simulink model "gm_mandelbrot_fpga"  (R2019b)
settings: Solver=FixedStepDiscrete  StartTime=0.0  StopTime=33.5e-3  FixedStep=0.5*Ts  RelTol=1e-3  EnableMultiTasking=on
undefined symbols (not defined in the file or in its folder): BUTTON_CLOCK_DIV, BUTTON_DEBOUNCE, BUTTON_POLLING, LUT_BLUE, LUT_GREEN, LUT_RED, MAX_ITERATIONS, PIXEL_TIME, TRASLATION_FACTOR, Ts, VGA_HORIZONTAL_BACK_PORCH, VGA_HORIZONTAL_FRONT_PORCH, VGA_HORIZONTAL_RESOLUTION, VGA_HORIZONTAL_SYNC, VGA_VERTICAL_BACK_PORCH, VGA_VERTICAL_FRONT_PORCH, VGA_VERTICAL_RESOLUTION, VGA_VERTICAL_SYNC, ZOOM_FACTOR
libraries: simulink x132, hdlsllib x20, visionsinks x1
(part 7 of 9)

== system gm_mandelbrot_fpga/mandelbrot_top/mandelbrot_core/mandelbroot_pipeline/mandelbroot_array_instance57 ==
  stop_in : Inport  OutDataTypeStr=boolean  PortDimensions=1  SampleTime=1.35e-08
  z_in : Inport  Port=2  OutDataTypeStr=fixdt(1, 18, 15)  PortDimensions=1  SampleTime=1.35e-08
      settings: SignalType=complex
  c_in : Inport  Port=3  OutDataTypeStr=fixdt(1, 18, 15)  PortDimensions=1  SampleTime=1.35e-08
      settings: SignalType=complex
  i_in : Inport  Port=4  OutDataTypeStr=fixdt(0, 7, 0)  PortDimensions=1  SampleTime=1.35e-08
  Add : Sum
  Add1 : Sum  Inputs=+-  OutDataTypeStr=Inherit: Same as first input
  Compare To Constant : simulink/Logic and Bit Operations/Compare To Constant  relop=>=  const=4  OutDataTypeStr=boolean
  Complex to Real-Imag : ComplexToRealImag
  Constant : Constant  OutDataTypeStr=uint8  SampleTime=-1
  Data Type Conversion2 : DataTypeConversion
  Gain : Gain  Gain=2  OutDataTypeStr=Inherit: Same as input  ParamDataTypeStr=Inherit: Same as input
  Logical Operator : Logic  Operator=OR  IconShape=distinctive  AllPortsSameDT=off  OutDataTypeStr=boolean
  Product1 : Product
  Product2 : Product
  Product3 : Product
  Real-Imag to Complex : RealImagToComplex
  Sum : Sum  Inputs=|++  OutDataTypeStr=Inherit: Same as first input
  Sum1 : Sum  Inputs=|++
  Switch : Switch  Criteria=u2 ~= 0
  stop_out : Outport  VectorParamsAs1DForOutWhenUnconnected=off
  z_out : Outport  Port=2  VectorParamsAs1DForOutWhenUnconnected=off
  c_out : Outport  Port=3  VectorParamsAs1DForOutWhenUnconnected=off
  i_out : Outport  Port=4  VectorParamsAs1DForOutWhenUnconnected=off
  wires:
  i_in/1 -> Switch/1, Sum1/1
  c_in/1 -> c_out/1, Sum/2
  z_in/1 -> Complex to Real-Imag/1
  stop_in/1 -> Logical Operator/1
  Add/1 -> Compare To Constant/1
  Add1/1 -> Real-Imag to Complex/1
  Compare To Constant/1 -> Logical Operator/2
  Complex to Real-Imag/2 -> Product3/2, Product2/1, Product2/2
  Complex to Real-Imag/1 -> Product3/1, Product1/1, Product1/2
  Constant/1 -> Sum1/2
  Data Type Conversion2/1 -> z_out/1
  Gain/1 -> Real-Imag to Complex/2
  Logical Operator/1 -> stop_out/1, Switch/2
  Product1/1 -> Add1/1, Add/1
  Product2/1 -> Add1/2, Add/2
  Product3/1 -> Gain/1
  Real-Imag to Complex/1 -> Sum/1
  Sum/1 -> Data Type Conversion2/1
  Sum1/1 -> Switch/3
  Switch/1 -> i_out/1

== system gm_mandelbrot_fpga/mandelbrot_top/mandelbrot_core/mandelbroot_pipeline/mandelbroot_array_instance58 ==
  stop_in : Inport  OutDataTypeStr=boolean  PortDimensions=1  SampleTime=1.35e-08
  z_in : Inport  Port=2  OutDataTypeStr=fixdt(1, 18, 15)  PortDimensions=1  SampleTime=1.35e-08
      settings: SignalType=complex
  c_in : Inport  Port=3  OutDataTypeStr=fixdt(1, 18, 15)  PortDimensions=1  SampleTime=1.35e-08
      settings: SignalType=complex
  i_in : Inport  Port=4  OutDataTypeStr=fixdt(0, 7, 0)  PortDimensions=1  SampleTime=1.35e-08
  Add : Sum
  Add1 : Sum  Inputs=+-  OutDataTypeStr=Inherit: Same as first input
  Compare To Constant : simulink/Logic and Bit Operations/Compare To Constant  relop=>=  const=4  OutDataTypeStr=boolean
  Complex to Real-Imag : ComplexToRealImag
  Constant : Constant  OutDataTypeStr=uint8  SampleTime=-1
  Data Type Conversion2 : DataTypeConversion
  Gain : Gain  Gain=2  OutDataTypeStr=Inherit: Same as input  ParamDataTypeStr=Inherit: Same as input
  Logical Operator : Logic  Operator=OR  IconShape=distinctive  AllPortsSameDT=off  OutDataTypeStr=boolean
  Product1 : Product
  Product2 : Product
  Product3 : Product
  Real-Imag to Complex : RealImagToComplex
  Sum : Sum  Inputs=|++  OutDataTypeStr=Inherit: Same as first input
  Sum1 : Sum  Inputs=|++
  Switch : Switch  Criteria=u2 ~= 0
  stop_out : Outport  VectorParamsAs1DForOutWhenUnconnected=off
  z_out : Outport  Port=2  VectorParamsAs1DForOutWhenUnconnected=off
  c_out : Outport  Port=3  VectorParamsAs1DForOutWhenUnconnected=off
  i_out : Outport  Port=4  VectorParamsAs1DForOutWhenUnconnected=off
  wires:
  i_in/1 -> Switch/1, Sum1/1
  c_in/1 -> c_out/1, Sum/2
  z_in/1 -> Complex to Real-Imag/1
  stop_in/1 -> Logical Operator/1
  Add/1 -> Compare To Constant/1
  Add1/1 -> Real-Imag to Complex/1
  Compare To Constant/1 -> Logical Operator/2
  Complex to Real-Imag/2 -> Product3/2, Product2/1, Product2/2
  Complex to Real-Imag/1 -> Product3/1, Product1/1, Product1/2
  Constant/1 -> Sum1/2
  Data Type Conversion2/1 -> z_out/1
  Gain/1 -> Real-Imag to Complex/2
  Logical Operator/1 -> stop_out/1, Switch/2
  Product1/1 -> Add1/1, Add/1
  Product2/1 -> Add1/2, Add/2
  Product3/1 -> Gain/1
  Real-Imag to Complex/1 -> Sum/1
  Sum/1 -> Data Type Conversion2/1
  Sum1/1 -> Switch/3
  Switch/1 -> i_out/1

== system gm_mandelbrot_fpga/mandelbrot_top/mandelbrot_core/mandelbroot_pipeline/mandelbroot_array_instance59 ==
  stop_in : Inport  OutDataTypeStr=boolean  PortDimensions=1  SampleTime=1.35e-08
  z_in : Inport  Port=2  OutDataTypeStr=fixdt(1, 18, 15)  PortDimensions=1  SampleTime=1.35e-08
      settings: SignalType=complex
  c_in : Inport  Port=3  OutDataTypeStr=fixdt(1, 18, 15)  PortDimensions=1  SampleTime=1.35e-08
      settings: SignalType=complex
  i_in : Inport  Port=4  OutDataTypeStr=fixdt(0, 7, 0)  PortDimensions=1  SampleTime=1.35e-08
  Add : Sum
  Add1 : Sum  Inputs=+-  OutDataTypeStr=Inherit: Same as first input
  Compare To Constant : simulink/Logic and Bit Operations/Compare To Constant  relop=>=  const=4  OutDataTypeStr=boolean
  Complex to Real-Imag : ComplexToRealImag
  Constant : Constant  OutDataTypeStr=uint8  SampleTime=-1
  Data Type Conversion2 : DataTypeConversion
  Gain : Gain  Gain=2  OutDataTypeStr=Inherit: Same as input  ParamDataTypeStr=Inherit: Same as input
  Logical Operator : Logic  Operator=OR  IconShape=distinctive  AllPortsSameDT=off  OutDataTypeStr=boolean
  Product1 : Product
  Product2 : Product
  Product3 : Product
  Real-Imag to Complex : RealImagToComplex
  Sum : Sum  Inputs=|++  OutDataTypeStr=Inherit: Same as first input
  Sum1 : Sum  Inputs=|++
  Switch : Switch  Criteria=u2 ~= 0
  stop_out : Outport  VectorParamsAs1DForOutWhenUnconnected=off
  z_out : Outport  Port=2  VectorParamsAs1DForOutWhenUnconnected=off
  c_out : Outport  Port=3  VectorParamsAs1DForOutWhenUnconnected=off
  i_out : Outport  Port=4  VectorParamsAs1DForOutWhenUnconnected=off
  wires:
  i_in/1 -> Switch/1, Sum1/1
  c_in/1 -> c_out/1, Sum/2
  z_in/1 -> Complex to Real-Imag/1
  stop_in/1 -> Logical Operator/1
  Add/1 -> Compare To Constant/1
  Add1/1 -> Real-Imag to Complex/1
  Compare To Constant/1 -> Logical Operator/2
  Complex to Real-Imag/2 -> Product3/2, Product2/1, Product2/2
  Complex to Real-Imag/1 -> Product3/1, Product1/1, Product1/2
  Constant/1 -> Sum1/2
  Data Type Conversion2/1 -> z_out/1
  Gain/1 -> Real-Imag to Complex/2
  Logical Operator/1 -> stop_out/1, Switch/2
  Product1/1 -> Add1/1, Add/1
  Product2/1 -> Add1/2, Add/2
  Product3/1 -> Gain/1
  Real-Imag to Complex/1 -> Sum/1
  Sum/1 -> Data Type Conversion2/1
  Sum1/1 -> Switch/3
  Switch/1 -> i_out/1

== system gm_mandelbrot_fpga/mandelbrot_top/mandelbrot_core/mandelbroot_pipeline/mandelbroot_array_instance6 ==
  stop_in : Inport  OutDataTypeStr=boolean  PortDimensions=1  SampleTime=1.35e-08
  z_in : Inport  Port=2  OutDataTypeStr=fixdt(1, 18, 15)  PortDimensions=1  SampleTime=1.35e-08
      settings: SignalType=complex
  c_in : Inport  Port=3  OutDataTypeStr=fixdt(1, 18, 15)  PortDimensions=1  SampleTime=1.35e-08
      settings: SignalType=complex
  i_in : Inport  Port=4  OutDataTypeStr=fixdt(0, 7, 0)  PortDimensions=1  SampleTime=1.35e-08
  Add : Sum
  Add1 : Sum  Inputs=+-  OutDataTypeStr=Inherit: Same as first input
  Compare To Constant : simulink/Logic and Bit Operations/Compare To Constant  relop=>=  const=4  OutDataTypeStr=boolean
  Complex to Real-Imag : ComplexToRealImag
  Constant : Constant  OutDataTypeStr=uint8  SampleTime=-1
  Data Type Conversion2 : DataTypeConversion
  Gain : Gain  Gain=2  OutDataTypeStr=Inherit: Same as input  ParamDataTypeStr=Inherit: Same as input
  Logical Operator : Logic  Operator=OR  IconShape=distinctive  AllPortsSameDT=off  OutDataTypeStr=boolean
  Product1 : Product
  Product2 : Product
  Product3 : Product
  Real-Imag to Complex : RealImagToComplex
  Sum : Sum  Inputs=|++  OutDataTypeStr=Inherit: Same as first input
  Sum1 : Sum  Inputs=|++
  Switch : Switch  Criteria=u2 ~= 0
  stop_out : Outport  VectorParamsAs1DForOutWhenUnconnected=off
  z_out : Outport  Port=2  VectorParamsAs1DForOutWhenUnconnected=off
  c_out : Outport  Port=3  VectorParamsAs1DForOutWhenUnconnected=off
  i_out : Outport  Port=4  VectorParamsAs1DForOutWhenUnconnected=off
  wires:
  i_in/1 -> Switch/1, Sum1/1
  c_in/1 -> c_out/1, Sum/2
  z_in/1 -> Complex to Real-Imag/1
  stop_in/1 -> Logical Operator/1
  Add/1 -> Compare To Constant/1
  Add1/1 -> Real-Imag to Complex/1
  Compare To Constant/1 -> Logical Operator/2
  Complex to Real-Imag/2 -> Product3/2, Product2/1, Product2/2
  Complex to Real-Imag/1 -> Product3/1, Product1/1, Product1/2
  Constant/1 -> Sum1/2
  Data Type Conversion2/1 -> z_out/1
  Gain/1 -> Real-Imag to Complex/2
  Logical Operator/1 -> stop_out/1, Switch/2
  Product1/1 -> Add1/1, Add/1
  Product2/1 -> Add1/2, Add/2
  Product3/1 -> Gain/1
  Real-Imag to Complex/1 -> Sum/1
  Sum/1 -> Data Type Conversion2/1
  Sum1/1 -> Switch/3
  Switch/1 -> i_out/1

== system gm_mandelbrot_fpga/mandelbrot_top/mandelbrot_core/mandelbroot_pipeline/mandelbroot_array_instance60 ==
  stop_in : Inport  OutDataTypeStr=boolean  PortDimensions=1  SampleTime=1.35e-08
  z_in : Inport  Port=2  OutDataTypeStr=fixdt(1, 18, 15)  PortDimensions=1  SampleTime=1.35e-08
      settings: SignalType=complex
  c_in : Inport  Port=3  OutDataTypeStr=fixdt(1, 18, 15)  PortDimensions=1  SampleTime=1.35e-08
      settings: SignalType=complex
  i_in : Inport  Port=4  OutDataTypeStr=fixdt(0, 7, 0)  PortDimensions=1  SampleTime=1.35e-08
  Add : Sum
  Add1 : Sum  Inputs=+-  OutDataTypeStr=Inherit: Same as first input
  Compare To Constant : simulink/Logic and Bit Operations/Compare To Constant  relop=>=  const=4  OutDataTypeStr=boolean
  Complex to Real-Imag : ComplexToRealImag
  Constant : Constant  OutDataTypeStr=uint8  SampleTime=-1
  Data Type Conversion2 : DataTypeConversion
  Gain : Gain  Gain=2  OutDataTypeStr=Inherit: Same as input  ParamDataTypeStr=Inherit: Same as input
  Logical Operator : Logic  Operator=OR  IconShape=distinctive  AllPortsSameDT=off  OutDataTypeStr=boolean
  Product1 : Product
  Product2 : Product
  Product3 : Product
  Real-Imag to Complex : RealImagToComplex
  Sum : Sum  Inputs=|++  OutDataTypeStr=Inherit: Same as first input
  Sum1 : Sum  Inputs=|++
  Switch : Switch  Criteria=u2 ~= 0
  stop_out : Outport  VectorParamsAs1DForOutWhenUnconnected=off
  z_out : Outport  Port=2  VectorParamsAs1DForOutWhenUnconnected=off
  c_out : Outport  Port=3  VectorParamsAs1DForOutWhenUnconnected=off
  i_out : Outport  Port=4  VectorParamsAs1DForOutWhenUnconnected=off
  wires:
  i_in/1 -> Switch/1, Sum1/1
  c_in/1 -> c_out/1, Sum/2
  z_in/1 -> Complex to Real-Imag/1
  stop_in/1 -> Logical Operator/1
  Add/1 -> Compare To Constant/1
  Add1/1 -> Real-Imag to Complex/1
  Compare To Constant/1 -> Logical Operator/2
  Complex to Real-Imag/2 -> Product3/2, Product2/1, Product2/2
  Complex to Real-Imag/1 -> Product3/1, Product1/1, Product1/2
  Constant/1 -> Sum1/2
  Data Type Conversion2/1 -> z_out/1
  Gain/1 -> Real-Imag to Complex/2
  Logical Operator/1 -> stop_out/1, Switch/2
  Product1/1 -> Add1/1, Add/1
  Product2/1 -> Add1/2, Add/2
  Product3/1 -> Gain/1
  Real-Imag to Complex/1 -> Sum/1
  Sum/1 -> Data Type Conversion2/1
  Sum1/1 -> Switch/3
  Switch/1 -> i_out/1

== system gm_mandelbrot_fpga/mandelbrot_top/mandelbrot_core/mandelbroot_pipeline/mandelbroot_array_instance61 ==
  stop_in : Inport  OutDataTypeStr=boolean  PortDimensions=1  SampleTime=1.35e-08
  z_in : Inport  Port=2  OutDataTypeStr=fixdt(1, 18, 15)  PortDimensions=1  SampleTime=1.35e-08
      settings: SignalType=complex
  c_in : Inport  Port=3  OutDataTypeStr=fixdt(1, 18, 15)  PortDimensions=1  SampleTime=1.35e-08
      settings: SignalType=complex
  i_in : Inport  Port=4  OutDataTypeStr=fixdt(0, 7, 0)  PortDimensions=1  SampleTime=1.35e-08
  Add : Sum
  Add1 : Sum  Inputs=+-  OutDataTypeStr=Inherit: Same as first input
  Compare To Constant : simulink/Logic and Bit Operations/Compare To Constant  relop=>=  const=4  OutDataTypeStr=boolean
  Complex to Real-Imag : ComplexToRealImag
  Constant : Constant  OutDataTypeStr=uint8  SampleTime=-1
  Data Type Conversion2 : DataTypeConversion
  Gain : Gain  Gain=2  OutDataTypeStr=Inherit: Same as input  ParamDataTypeStr=Inherit: Same as input
  Logical Operator : Logic  Operator=OR  IconShape=distinctive  AllPortsSameDT=off  OutDataTypeStr=boolean
  Product1 : Product
  Product2 : Product
  Product3 : Product
  Real-Imag to Complex : RealImagToComplex
  Sum : Sum  Inputs=|++  OutDataTypeStr=Inherit: Same as first input
  Sum1 : Sum  Inputs=|++
  Switch : Switch  Criteria=u2 ~= 0
  stop_out : Outport  VectorParamsAs1DForOutWhenUnconnected=off
  z_out : Outport  Port=2  VectorParamsAs1DForOutWhenUnconnected=off
  c_out : Outport  Port=3  VectorParamsAs1DForOutWhenUnconnected=off
  i_out : Outport  Port=4  VectorParamsAs1DForOutWhenUnconnected=off
  wires:
  i_in/1 -> Switch/1, Sum1/1
  c_in/1 -> c_out/1, Sum/2
  z_in/1 -> Complex to Real-Imag/1
  stop_in/1 -> Logical Operator/1
  Add/1 -> Compare To Constant/1
  Add1/1 -> Real-Imag to Complex/1
  Compare To Constant/1 -> Logical Operator/2
  Complex to Real-Imag/2 -> Product3/2, Product2/1, Product2/2
  Complex to Real-Imag/1 -> Product3/1, Product1/1, Product1/2
  Constant/1 -> Sum1/2
  Data Type Conversion2/1 -> z_out/1
  Gain/1 -> Real-Imag to Complex/2
  Logical Operator/1 -> stop_out/1, Switch/2
  Product1/1 -> Add1/1, Add/1
  Product2/1 -> Add1/2, Add/2
  Product3/1 -> Gain/1
  Real-Imag to Complex/1 -> Sum/1
  Sum/1 -> Data Type Conversion2/1
  Sum1/1 -> Switch/3
  Switch/1 -> i_out/1

== system gm_mandelbrot_fpga/mandelbrot_top/mandelbrot_core/mandelbroot_pipeline/mandelbroot_array_instance62 ==
  stop_in : Inport  OutDataTypeStr=boolean  PortDimensions=1  SampleTime=1.35e-08
  z_in : Inport  Port=2  OutDataTypeStr=fixdt(1, 18, 15)  PortDimensions=1  SampleTime=1.35e-08
      settings: SignalType=complex
  c_in : Inport  Port=3  OutDataTypeStr=fixdt(1, 18, 15)  PortDimensions=1  SampleTime=1.35e-08
      settings: SignalType=complex
  i_in : Inport  Port=4  OutDataTypeStr=fixdt(0, 7, 0)  PortDimensions=1  SampleTime=1.35e-08
  Add : Sum
  Add1 : Sum  Inputs=+-  OutDataTypeStr=Inherit: Same as first input
  Compare To Constant : simulink/Logic and Bit Operations/Compare To Constant  relop=>=  const=4  OutDataTypeStr=boolean
  Complex to Real-Imag : ComplexToRealImag
  Constant : Constant  OutDataTypeStr=uint8  SampleTime=-1
  Data Type Conversion2 : DataTypeConversion
  Gain : Gain  Gain=2  OutDataTypeStr=Inherit: Same as input  ParamDataTypeStr=Inherit: Same as input
  Logical Operator : Logic  Operator=OR  IconShape=distinctive  AllPortsSameDT=off  OutDataTypeStr=boolean
  Product1 : Product
  Product2 : Product
  Product3 : Product
  Real-Imag to Complex : RealImagToComplex
  Sum : Sum  Inputs=|++  OutDataTypeStr=Inherit: Same as first input
  Sum1 : Sum  Inputs=|++
  Switch : Switch  Criteria=u2 ~= 0
  stop_out : Outport  VectorParamsAs1DForOutWhenUnconnected=off
  z_out : Outport  Port=2  VectorParamsAs1DForOutWhenUnconnected=off
  c_out : Outport  Port=3  VectorParamsAs1DForOutWhenUnconnected=off
  i_out : Outport  Port=4  VectorParamsAs1DForOutWhenUnconnected=off
  wires:
  i_in/1 -> Switch/1, Sum1/1
  c_in/1 -> c_out/1, Sum/2
  z_in/1 -> Complex to Real-Imag/1
  stop_in/1 -> Logical Operator/1
  Add/1 -> Compare To Constant/1
  Add1/1 -> Real-Imag to Complex/1
  Compare To Constant/1 -> Logical Operator/2
  Complex to Real-Imag/2 -> Product3/2, Product2/1, Product2/2
  Complex to Real-Imag/1 -> Product3/1, Product1/1, Product1/2
  Constant/1 -> Sum1/2
  Data Type Conversion2/1 -> z_out/1
  Gain/1 -> Real-Imag to Complex/2
  Logical Operator/1 -> stop_out/1, Switch/2
  Product1/1 -> Add1/1, Add/1
  Product2/1 -> Add1/2, Add/2
  Product3/1 -> Gain/1
  Real-Imag to Complex/1 -> Sum/1
  Sum/1 -> Data Type Conversion2/1
  Sum1/1 -> Switch/3
  Switch/1 -> i_out/1

== system gm_mandelbrot_fpga/mandelbrot_top/mandelbrot_core/mandelbroot_pipeline/mandelbroot_array_instance63 ==
  stop_in : Inport  OutDataTypeStr=boolean  PortDimensions=1  SampleTime=1.35e-08
  z_in : Inport  Port=2  OutDataTypeStr=fixdt(1, 18, 15)  PortDimensions=1  SampleTime=1.35e-08
      settings: SignalType=complex
  c_in : Inport  Port=3  OutDataTypeStr=fixdt(1, 18, 15)  PortDimensions=1  SampleTime=1.35e-08
      settings: SignalType=complex
  i_in : Inport  Port=4  OutDataTypeStr=fixdt(0, 7, 0)  PortDimensions=1  SampleTime=1.35e-08
  Add : Sum
  Add1 : Sum  Inputs=+-  OutDataTypeStr=Inherit: Same as first input
  Compare To Constant : simulink/Logic and Bit Operations/Compare To Constant  relop=>=  const=4  OutDataTypeStr=boolean
  Complex to Real-Imag : ComplexToRealImag
  Constant : Constant  OutDataTypeStr=uint8  SampleTime=-1
  Data Type Conversion2 : DataTypeConversion
  Gain : Gain  Gain=2  OutDataTypeStr=Inherit: Same as input  ParamDataTypeStr=Inherit: Same as input
  Logical Operator : Logic  Operator=OR  IconShape=distinctive  AllPortsSameDT=off  OutDataTypeStr=boolean
  Product1 : Product
  Product2 : Product
  Product3 : Product
  Real-Imag to Complex : RealImagToComplex
  Sum : Sum  Inputs=|++  OutDataTypeStr=Inherit: Same as first input
  Sum1 : Sum  Inputs=|++
  Switch : Switch  Criteria=u2 ~= 0
  stop_out : Outport  VectorParamsAs1DForOutWhenUnconnected=off
  z_out : Outport  Port=2  VectorParamsAs1DForOutWhenUnconnected=off
  c_out : Outport  Port=3  VectorParamsAs1DForOutWhenUnconnected=off
  i_out : Outport  Port=4  VectorParamsAs1DForOutWhenUnconnected=off
  wires:
  i_in/1 -> Switch/1, Sum1/1
  c_in/1 -> c_out/1, Sum/2
  z_in/1 -> Complex to Real-Imag/1
  stop_in/1 -> Logical Operator/1
  Add/1 -> Compare To Constant/1
  Add1/1 -> Real-Imag to Complex/1
  Compare To Constant/1 -> Logical Operator/2
  Complex to Real-Imag/2 -> Product3/2, Product2/1, Product2/2
  Complex to Real-Imag/1 -> Product3/1, Product1/1, Product1/2
  Constant/1 -> Sum1/2
  Data Type Conversion2/1 -> z_out/1
  Gain/1 -> Real-Imag to Complex/2
  Logical Operator/1 -> stop_out/1, Switch/2
  Product1/1 -> Add1/1, Add/1
  Product2/1 -> Add1/2, Add/2
  Product3/1 -> Gain/1
  Real-Imag to Complex/1 -> Sum/1
  Sum/1 -> Data Type Conversion2/1
  Sum1/1 -> Switch/3
  Switch/1 -> i_out/1

== system gm_mandelbrot_fpga/mandelbrot_top/mandelbrot_core/mandelbroot_pipeline/mandelbroot_array_instance64 ==
  stop_in : Inport  OutDataTypeStr=boolean  PortDimensions=1  SampleTime=1.35e-08
  z_in : Inport  Port=2  OutDataTypeStr=fixdt(1, 18, 15)  PortDimensions=1  SampleTime=1.35e-08
      settings: SignalType=complex
  c_in : Inport  Port=3  OutDataTypeStr=fixdt(1, 18, 15)  PortDimensions=1  SampleTime=1.35e-08
      settings: SignalType=complex
  i_in : Inport  Port=4  OutDataTypeStr=fixdt(0, 7, 0)  PortDimensions=1  SampleTime=1.35e-08
  Add : Sum
  Add1 : Sum  Inputs=+-  OutDataTypeStr=Inherit: Same as first input
  Compare To Constant : simulink/Logic and Bit Operations/Compare To Constant  relop=>=  const=4  OutDataTypeStr=boolean
  Complex to Real-Imag : ComplexToRealImag
  Constant : Constant  OutDataTypeStr=uint8  SampleTime=-1
  Data Type Conversion2 : DataTypeConversion
  Gain : Gain  Gain=2  OutDataTypeStr=Inherit: Same as input  ParamDataTypeStr=Inherit: Same as input
  Logical Operator : Logic  Operator=OR  IconShape=distinctive  AllPortsSameDT=off  OutDataTypeStr=boolean
  Product1 : Product
  Product2 : Product
  Product3 : Product
  Real-Imag to Complex : RealImagToComplex
  Sum : Sum  Inputs=|++  OutDataTypeStr=Inherit: Same as first input
  Sum1 : Sum  Inputs=|++
  Switch : Switch  Criteria=u2 ~= 0
  stop_out : Outport  VectorParamsAs1DForOutWhenUnconnected=off
  z_out : Outport  Port=2  VectorParamsAs1DForOutWhenUnconnected=off
  c_out : Outport  Port=3  VectorParamsAs1DForOutWhenUnconnected=off
  i_out : Outport  Port=4  VectorParamsAs1DForOutWhenUnconnected=off
  wires:
  i_in/1 -> Switch/1, Sum1/1
  c_in/1 -> c_out/1, Sum/2
  z_in/1 -> Complex to Real-Imag/1
  stop_in/1 -> Logical Operator/1
  Add/1 -> Compare To Constant/1
  Add1/1 -> Real-Imag to Complex/1
  Compare To Constant/1 -> Logical Operator/2
  Complex to Real-Imag/2 -> Product3/2, Product2/1, Product2/2
  Complex to Real-Imag/1 -> Product3/1, Product1/1, Product1/2
  Constant/1 -> Sum1/2
  Data Type Conversion2/1 -> z_out/1
  Gain/1 -> Real-Imag to Complex/2
  Logical Operator/1 -> stop_out/1, Switch/2
  Product1/1 -> Add1/1, Add/1
  Product2/1 -> Add1/2, Add/2
  Product3/1 -> Gain/1
  Real-Imag to Complex/1 -> Sum/1
  Sum/1 -> Data Type Conversion2/1
  Sum1/1 -> Switch/3
  Switch/1 -> i_out/1

== system gm_mandelbrot_fpga/mandelbrot_top/mandelbrot_core/mandelbroot_pipeline/mandelbroot_array_instance65 ==
  stop_in : Inport  OutDataTypeStr=boolean  PortDimensions=1  SampleTime=1.35e-08
  z_in : Inport  Port=2  OutDataTypeStr=fixdt(1, 18, 15)  PortDimensions=1  SampleTime=1.35e-08
      settings: SignalType=complex
  c_in : Inport  Port=3  OutDataTypeStr=fixdt(1, 18, 15)  PortDimensions=1  SampleTime=1.35e-08
      settings: SignalType=complex
  i_in : Inport  Port=4  OutDataTypeStr=fixdt(0, 7, 0)  PortDimensions=1  SampleTime=1.35e-08
  Add : Sum
  Add1 : Sum  Inputs=+-  OutDataTypeStr=Inherit: Same as first input
  Compare To Constant : simulink/Logic and Bit Operations/Compare To Constant  relop=>=  const=4  OutDataTypeStr=boolean
  Complex to Real-Imag : ComplexToRealImag
  Constant : Constant  OutDataTypeStr=uint8  SampleTime=-1
  Data Type Conversion2 : DataTypeConversion
  Gain : Gain  Gain=2  OutDataTypeStr=Inherit: Same as input  ParamDataTypeStr=Inherit: Same as input
  Logical Operator : Logic  Operator=OR  IconShape=distinctive  AllPortsSameDT=off  OutDataTypeStr=boolean
  Product1 : Product
  Product2 : Product
  Product3 : Product
  Real-Imag to Complex : RealImagToComplex
  Sum : Sum  Inputs=|++  OutDataTypeStr=Inherit: Same as first input
  Sum1 : Sum  Inputs=|++
  Switch : Switch  Criteria=u2 ~= 0
  stop_out : Outport  VectorParamsAs1DForOutWhenUnconnected=off
  z_out : Outport  Port=2  VectorParamsAs1DForOutWhenUnconnected=off
  c_out : Outport  Port=3  VectorParamsAs1DForOutWhenUnconnected=off
  i_out : Outport  Port=4  VectorParamsAs1DForOutWhenUnconnected=off
  wires:
  i_in/1 -> Switch/1, Sum1/1
  c_in/1 -> c_out/1, Sum/2
  z_in/1 -> Complex to Real-Imag/1
  stop_in/1 -> Logical Operator/1
  Add/1 -> Compare To Constant/1
  Add1/1 -> Real-Imag to Complex/1
  Compare To Constant/1 -> Logical Operator/2
  Complex to Real-Imag/2 -> Product3/2, Product2/1, Product2/2
  Complex to Real-Imag/1 -> Product3/1, Product1/1, Product1/2
  Constant/1 -> Sum1/2
  Data Type Conversion2/1 -> z_out/1
  Gain/1 -> Real-Imag to Complex/2
  Logical Operator/1 -> stop_out/1, Switch/2
  Product1/1 -> Add1/1, Add/1
  Product2/1 -> Add1/2, Add/2
  Product3/1 -> Gain/1
  Real-Imag to Complex/1 -> Sum/1
  Sum/1 -> Data Type Conversion2/1
  Sum1/1 -> Switch/3
  Switch/1 -> i_out/1

== system gm_mandelbrot_fpga/mandelbrot_top/mandelbrot_core/mandelbroot_pipeline/mandelbroot_array_instance66 ==
  stop_in : Inport  OutDataTypeStr=boolean  PortDimensions=1  SampleTime=1.35e-08
  z_in : Inport  Port=2  OutDataTypeStr=fixdt(1, 18, 15)  PortDimensions=1  SampleTime=1.35e-08
      settings: SignalType=complex
  c_in : Inport  Port=3  OutDataTypeStr=fixdt(1, 18, 15)  PortDimensions=1  SampleTime=1.35e-08
      settings: SignalType=complex
  i_in : Inport  Port=4  OutDataTypeStr=fixdt(0, 7, 0)  PortDimensions=1  SampleTime=1.35e-08
  Add : Sum
  Add1 : Sum  Inputs=+-  OutDataTypeStr=Inherit: Same as first input
  Compare To Constant : simulink/Logic and Bit Operations/Compare To Constant  relop=>=  const=4  OutDataTypeStr=boolean
  Complex to Real-Imag : ComplexToRealImag
  Constant : Constant  OutDataTypeStr=uint8  SampleTime=-1
  Data Type Conversion2 : DataTypeConversion
  Gain : Gain  Gain=2  OutDataTypeStr=Inherit: Same as input  ParamDataTypeStr=Inherit: Same as input
  Logical Operator : Logic  Operator=OR  IconShape=distinctive  AllPortsSameDT=off  OutDataTypeStr=boolean
  Product1 : Product
  Product2 : Product
  Product3 : Product
  Real-Imag to Complex : RealImagToComplex
  Sum : Sum  Inputs=|++  OutDataTypeStr=Inherit: Same as first input
  Sum1 : Sum  Inputs=|++
  Switch : Switch  Criteria=u2 ~= 0
  stop_out : Outport  VectorParamsAs1DForOutWhenUnconnected=off
  z_out : Outport  Port=2  VectorParamsAs1DForOutWhenUnconnected=off
  c_out : Outport  Port=3  VectorParamsAs1DForOutWhenUnconnected=off
  i_out : Outport  Port=4  VectorParamsAs1DForOutWhenUnconnected=off
  wires:
  i_in/1 -> Switch/1, Sum1/1
  c_in/1 -> c_out/1, Sum/2
  z_in/1 -> Complex to Real-Imag/1
  stop_in/1 -> Logical Operator/1
  Add/1 -> Compare To Constant/1
  Add1/1 -> Real-Imag to Complex/1
  Compare To Constant/1 -> Logical Operator/2
  Complex to Real-Imag/2 -> Product3/2, Product2/1, Product2/2
  Complex to Real-Imag/1 -> Product3/1, Product1/1, Product1/2
  Constant/1 -> Sum1/2
  Data Type Conversion2/1 -> z_out/1
  Gain/1 -> Real-Imag to Complex/2
  Logical Operator/1 -> stop_out/1, Switch/2
  Product1/1 -> Add1/1, Add/1
  Product2/1 -> Add1/2, Add/2
  Product3/1 -> Gain/1
  Real-Imag to Complex/1 -> Sum/1
  Sum/1 -> Data Type Conversion2/1
  Sum1/1 -> Switch/3
  Switch/1 -> i_out/1

== system gm_mandelbrot_fpga/mandelbrot_top/mandelbrot_core/mandelbroot_pipeline/mandelbroot_array_instance67 ==
  stop_in : Inport  OutDataTypeStr=boolean  PortDimensions=1  SampleTime=1.35e-08
  z_in : Inport  Port=2  OutDataTypeStr=fixdt(1, 18, 15)  PortDimensions=1  SampleTime=1.35e-08
      settings: SignalType=complex
  c_in : Inport  Port=3  OutDataTypeStr=fixdt(1, 18, 15)  PortDimensions=1  SampleTime=1.35e-08
      settings: SignalType=complex
  i_in : Inport  Port=4  OutDataTypeStr=fixdt(0, 7, 0)  PortDimensions=1  SampleTime=1.35e-08
  Add : Sum
  Add1 : Sum  Inputs=+-  OutDataTypeStr=Inherit: Same as first input
  Compare To Constant : simulink/Logic and Bit Operations/Compare To Constant  relop=>=  const=4  OutDataTypeStr=boolean
  Complex to Real-Imag : ComplexToRealImag
  Constant : Constant  OutDataTypeStr=uint8  SampleTime=-1
  Data Type Conversion2 : DataTypeConversion
  Gain : Gain  Gain=2  OutDataTypeStr=Inherit: Same as input  ParamDataTypeStr=Inherit: Same as input
  Logical Operator : Logic  Operator=OR  IconShape=distinctive  AllPortsSameDT=off  OutDataTypeStr=boolean
  Product1 : Product
  Product2 : Product
  Product3 : Product
  Real-Imag to Complex : RealImagToComplex
  Sum : Sum  Inputs=|++  OutDataTypeStr=Inherit: Same as first input
  Sum1 : Sum  Inputs=|++
  Switch : Switch  Criteria=u2 ~= 0
  stop_out : Outport  VectorParamsAs1DForOutWhenUnconnected=off
  z_out : Outport  Port=2  VectorParamsAs1DForOutWhenUnconnected=off
  c_out : Outport  Port=3  VectorParamsAs1DForOutWhenUnconnected=off
  i_out : Outport  Port=4  VectorParamsAs1DForOutWhenUnconnected=off
  wires:
  i_in/1 -> Switch/1, Sum1/1
  c_in/1 -> c_out/1, Sum/2
  z_in/1 -> Complex to Real-Imag/1
  stop_in/1 -> Logical Operator/1
  Add/1 -> Compare To Constant/1
  Add1/1 -> Real-Imag to Complex/1
  Compare To Constant/1 -> Logical Operator/2
  Complex to Real-Imag/2 -> Product3/2, Product2/1, Product2/2
  Complex to Real-Imag/1 -> Product3/1, Product1/1, Product1/2
  Constant/1 -> Sum1/2
  Data Type Conversion2/1 -> z_out/1
  Gain/1 -> Real-Imag to Complex/2
  Logical Operator/1 -> stop_out/1, Switch/2
  Product1/1 -> Add1/1, Add/1
  Product2/1 -> Add1/2, Add/2
  Product3/1 -> Gain/1
  Real-Imag to Complex/1 -> Sum/1
  Sum/1 -> Data Type Conversion2/1
  Sum1/1 -> Switch/3
  Switch/1 -> i_out/1

== system gm_mandelbrot_fpga/mandelbrot_top/mandelbrot_core/mandelbroot_pipeline/mandelbroot_array_instance68 ==
  stop_in : Inport  OutDataTypeStr=boolean  PortDimensions=1  SampleTime=1.35e-08
  z_in : Inport  Port=2  OutDataTypeStr=fixdt(1, 18, 15)  PortDimensions=1  SampleTime=1.35e-08
      settings: SignalType=complex
  c_in : Inport  Port=3  OutDataTypeStr=fixdt(1, 18, 15)  PortDimensions=1  SampleTime=1.35e-08
      settings: SignalType=complex
  i_in : Inport  Port=4  OutDataTypeStr=fixdt(0, 7, 0)  PortDimensions=1  SampleTime=1.35e-08
  Add : Sum
  Add1 : Sum  Inputs=+-  OutDataTypeStr=Inherit: Same as first input
  Compare To Constant : simulink/Logic and Bit Operations/Compare To Constant  relop=>=  const=4  OutDataTypeStr=boolean
  Complex to Real-Imag : ComplexToRealImag
  Constant : Constant  OutDataTypeStr=uint8  SampleTime=-1
  Data Type Conversion2 : DataTypeConversion
  Gain : Gain  Gain=2  OutDataTypeStr=Inherit: Same as input  ParamDataTypeStr=Inherit: Same as input
  Logical Operator : Logic  Operator=OR  IconShape=distinctive  AllPortsSameDT=off  OutDataTypeStr=boolean
  Product1 : Product
  Product2 : Product
  Product3 : Product
  Real-Imag to Complex : RealImagToComplex
  Sum : Sum  Inputs=|++  OutDataTypeStr=Inherit: Same as first input
  Sum1 : Sum  Inputs=|++
  Switch : Switch  Criteria=u2 ~= 0
  stop_out : Outport  VectorParamsAs1DForOutWhenUnconnected=off
  z_out : Outport  Port=2  VectorParamsAs1DForOutWhenUnconnected=off
  c_out : Outport  Port=3  VectorParamsAs1DForOutWhenUnconnected=off
  i_out : Outport  Port=4  VectorParamsAs1DForOutWhenUnconnected=off
  wires:
  i_in/1 -> Switch/1, Sum1/1
  c_in/1 -> c_out/1, Sum/2
  z_in/1 -> Complex to Real-Imag/1
  stop_in/1 -> Logical Operator/1
  Add/1 -> Compare To Constant/1
  Add1/1 -> Real-Imag to Complex/1
  Compare To Constant/1 -> Logical Operator/2
  Complex to Real-Imag/2 -> Product3/2, Product2/1, Product2/2
  Complex to Real-Imag/1 -> Product3/1, Product1/1, Product1/2
  Constant/1 -> Sum1/2
  Data Type Conversion2/1 -> z_out/1
  Gain/1 -> Real-Imag to Complex/2
  Logical Operator/1 -> stop_out/1, Switch/2
  Product1/1 -> Add1/1, Add/1
  Product2/1 -> Add1/2, Add/2
  Product3/1 -> Gain/1
  Real-Imag to Complex/1 -> Sum/1
  Sum/1 -> Data Type Conversion2/1
  Sum1/1 -> Switch/3
  Switch/1 -> i_out/1

== system gm_mandelbrot_fpga/mandelbrot_top/mandelbrot_core/mandelbroot_pipeline/mandelbroot_array_instance69 ==
  stop_in : Inport  OutDataTypeStr=boolean  PortDimensions=1  SampleTime=1.35e-08
  z_in : Inport  Port=2  OutDataTypeStr=fixdt(1, 18, 15)  PortDimensions=1  SampleTime=1.35e-08
      settings: SignalType=complex
  c_in : Inport  Port=3  OutDataTypeStr=fixdt(1, 18, 15)  PortDimensions=1  SampleTime=1.35e-08
      settings: SignalType=complex
  i_in : Inport  Port=4  OutDataTypeStr=fixdt(0, 7, 0)  PortDimensions=1  SampleTime=1.35e-08
  Add : Sum
  Add1 : Sum  Inputs=+-  OutDataTypeStr=Inherit: Same as first input
  Compare To Constant : simulink/Logic and Bit Operations/Compare To Constant  relop=>=  const=4  OutDataTypeStr=boolean
  Complex to Real-Imag : ComplexToRealImag
  Constant : Constant  OutDataTypeStr=uint8  SampleTime=-1
  Data Type Conversion2 : DataTypeConversion
  Gain : Gain  Gain=2  OutDataTypeStr=Inherit: Same as input  ParamDataTypeStr=Inherit: Same as input
  Logical Operator : Logic  Operator=OR  IconShape=distinctive  AllPortsSameDT=off  OutDataTypeStr=boolean
  Product1 : Product
  Product2 : Product
  Product3 : Product
  Real-Imag to Complex : RealImagToComplex
  Sum : Sum  Inputs=|++  OutDataTypeStr=Inherit: Same as first input
  Sum1 : Sum  Inputs=|++
  Switch : Switch  Criteria=u2 ~= 0
  stop_out : Outport  VectorParamsAs1DForOutWhenUnconnected=off
  z_out : Outport  Port=2  VectorParamsAs1DForOutWhenUnconnected=off
  c_out : Outport  Port=3  VectorParamsAs1DForOutWhenUnconnected=off
  i_out : Outport  Port=4  VectorParamsAs1DForOutWhenUnconnected=off
  wires:
  i_in/1 -> Switch/1, Sum1/1
  c_in/1 -> c_out/1, Sum/2
  z_in/1 -> Complex to Real-Imag/1
  stop_in/1 -> Logical Operator/1
  Add/1 -> Compare To Constant/1
  Add1/1 -> Real-Imag to Complex/1
  Compare To Constant/1 -> Logical Operator/2
  Complex to Real-Imag/2 -> Product3/2, Product2/1, Product2/2
  Complex to Real-Imag/1 -> Product3/1, Product1/1, Product1/2
  Constant/1 -> Sum1/2
  Data Type Conversion2/1 -> z_out/1
  Gain/1 -> Real-Imag to Complex/2
  Logical Operator/1 -> stop_out/1, Switch/2
  Product1/1 -> Add1/1, Add/1
  Product2/1 -> Add1/2, Add/2
  Product3/1 -> Gain/1
  Real-Imag to Complex/1 -> Sum/1
  Sum/1 -> Data Type Conversion2/1
  Sum1/1 -> Switch/3
  Switch/1 -> i_out/1

== system gm_mandelbrot_fpga/mandelbrot_top/mandelbrot_core/mandelbroot_pipeline/mandelbroot_array_instance7 ==
  stop_in : Inport  OutDataTypeStr=boolean  PortDimensions=1  SampleTime=1.35e-08
  z_in : Inport  Port=2  OutDataTypeStr=fixdt(1, 18, 15)  PortDimensions=1  SampleTime=1.35e-08
      settings: SignalType=complex
  c_in : Inport  Port=3  OutDataTypeStr=fixdt(1, 18, 15)  PortDimensions=1  SampleTime=1.35e-08
      settings: SignalType=complex
  i_in : Inport  Port=4  OutDataTypeStr=fixdt(0, 7, 0)  PortDimensions=1  SampleTime=1.35e-08
  Add : Sum
  Add1 : Sum  Inputs=+-  OutDataTypeStr=Inherit: Same as first input
  Compare To Constant : simulink/Logic and Bit Operations/Compare To Constant  relop=>=  const=4  OutDataTypeStr=boolean
  Complex to Real-Imag : ComplexToRealImag
  Constant : Constant  OutDataTypeStr=uint8  SampleTime=-1
  Data Type Conversion2 : DataTypeConversion
  Gain : Gain  Gain=2  OutDataTypeStr=Inherit: Same as input  ParamDataTypeStr=Inherit: Same as input
  Logical Operator : Logic  Operator=OR  IconShape=distinctive  AllPortsSameDT=off  OutDataTypeStr=boolean
  Product1 : Product
  Product2 : Product
  Product3 : Product
  Real-Imag to Complex : RealImagToComplex
  Sum : Sum  Inputs=|++  OutDataTypeStr=Inherit: Same as first input
  Sum1 : Sum  Inputs=|++
  Switch : Switch  Criteria=u2 ~= 0
  stop_out : Outport  VectorParamsAs1DForOutWhenUnconnected=off
  z_out : Outport  Port=2  VectorParamsAs1DForOutWhenUnconnected=off
  c_out : Outport  Port=3  VectorParamsAs1DForOutWhenUnconnected=off
  i_out : Outport  Port=4  VectorParamsAs1DForOutWhenUnconnected=off
  wires:
  i_in/1 -> Switch/1, Sum1/1
  c_in/1 -> c_out/1, Sum/2
  z_in/1 -> Complex to Real-Imag/1
  stop_in/1 -> Logical Operator/1
  Add/1 -> Compare To Constant/1
  Add1/1 -> Real-Imag to Complex/1
  Compare To Constant/1 -> Logical Operator/2
  Complex to Real-Imag/2 -> Product3/2, Product2/1, Product2/2
  Complex to Real-Imag/1 -> Product3/1, Product1/1, Product1/2
  Constant/1 -> Sum1/2
  Data Type Conversion2/1 -> z_out/1
  Gain/1 -> Real-Imag to Complex/2
  Logical Operator/1 -> stop_out/1, Switch/2
  Product1/1 -> Add1/1, Add/1
  Product2/1 -> Add1/2, Add/2
  Product3/1 -> Gain/1
  Real-Imag to Complex/1 -> Sum/1
  Sum/1 -> Data Type Conversion2/1
  Sum1/1 -> Switch/3
  Switch/1 -> i_out/1

== system gm_mandelbrot_fpga/mandelbrot_top/mandelbrot_core/mandelbroot_pipeline/mandelbroot_array_instance70 ==
  stop_in : Inport  OutDataTypeStr=boolean  PortDimensions=1  SampleTime=1.35e-08
  z_in : Inport  Port=2  OutDataTypeStr=fixdt(1, 18, 15)  PortDimensions=1  SampleTime=1.35e-08
      settings: SignalType=complex
  c_in : Inport  Port=3  OutDataTypeStr=fixdt(1, 18, 15)  PortDimensions=1  SampleTime=1.35e-08
      settings: SignalType=complex
  i_in : Inport  Port=4  OutDataTypeStr=fixdt(0, 7, 0)  PortDimensions=1  SampleTime=1.35e-08
  Add : Sum
  Add1 : Sum  Inputs=+-  OutDataTypeStr=Inherit: Same as first input
  Compare To Constant : simulink/Logic and Bit Operations/Compare To Constant  relop=>=  const=4  OutDataTypeStr=boolean
  Complex to Real-Imag : ComplexToRealImag
  Constant : Constant  OutDataTypeStr=uint8  SampleTime=-1
  Data Type Conversion2 : DataTypeConversion
  Gain : Gain  Gain=2  OutDataTypeStr=Inherit: Same as input  ParamDataTypeStr=Inherit: Same as input
  Logical Operator : Logic  Operator=OR  IconShape=distinctive  AllPortsSameDT=off  OutDataTypeStr=boolean
  Product1 : Product
  Product2 : Product
  Product3 : Product
  Real-Imag to Complex : RealImagToComplex
  Sum : Sum  Inputs=|++  OutDataTypeStr=Inherit: Same as first input
  Sum1 : Sum  Inputs=|++
  Switch : Switch  Criteria=u2 ~= 0
  stop_out : Outport  VectorParamsAs1DForOutWhenUnconnected=off
  z_out : Outport  Port=2  VectorParamsAs1DForOutWhenUnconnected=off
  c_out : Outport  Port=3  VectorParamsAs1DForOutWhenUnconnected=off
  i_out : Outport  Port=4  VectorParamsAs1DForOutWhenUnconnected=off
  wires:
  i_in/1 -> Switch/1, Sum1/1
  c_in/1 -> c_out/1, Sum/2
  z_in/1 -> Complex to Real-Imag/1
  stop_in/1 -> Logical Operator/1
  Add/1 -> Compare To Constant/1
  Add1/1 -> Real-Imag to Complex/1
  Compare To Constant/1 -> Logical Operator/2
  Complex to Real-Imag/2 -> Product3/2, Product2/1, Product2/2
  Complex to Real-Imag/1 -> Product3/1, Product1/1, Product1/2
  Constant/1 -> Sum1/2
  Data Type Conversion2/1 -> z_out/1
  Gain/1 -> Real-Imag to Complex/2
  Logical Operator/1 -> stop_out/1, Switch/2
  Product1/1 -> Add1/1, Add/1
  Product2/1 -> Add1/2, Add/2
  Product3/1 -> Gain/1
  Real-Imag to Complex/1 -> Sum/1
  Sum/1 -> Data Type Conversion2/1
  Sum1/1 -> Switch/3
  Switch/1 -> i_out/1

== system gm_mandelbrot_fpga/mandelbrot_top/mandelbrot_core/mandelbroot_pipeline/mandelbroot_array_instance71 ==
  stop_in : Inport  OutDataTypeStr=boolean  PortDimensions=1  SampleTime=1.35e-08
  z_in : Inport  Port=2  OutDataTypeStr=fixdt(1, 18, 15)  PortDimensions=1  SampleTime=1.35e-08
      settings: SignalType=complex
  c_in : Inport  Port=3  OutDataTypeStr=fixdt(1, 18, 15)  PortDimensions=1  SampleTime=1.35e-08
      settings: SignalType=complex
  i_in : Inport  Port=4  OutDataTypeStr=fixdt(0, 7, 0)  PortDimensions=1  SampleTime=1.35e-08
  Add : Sum
  Add1 : Sum  Inputs=+-  OutDataTypeStr=Inherit: Same as first input
  Compare To Constant : simulink/Logic and Bit Operations/Compare To Constant  relop=>=  const=4  OutDataTypeStr=boolean
  Complex to Real-Imag : ComplexToRealImag
  Constant : Constant  OutDataTypeStr=uint8  SampleTime=-1
  Data Type Conversion2 : DataTypeConversion
  Gain : Gain  Gain=2  OutDataTypeStr=Inherit: Same as input  ParamDataTypeStr=Inherit: Same as input
  Logical Operator : Logic  Operator=OR  IconShape=distinctive  AllPortsSameDT=off  OutDataTypeStr=boolean
  Product1 : Product
  Product2 : Product
  Product3 : Product
  Real-Imag to Complex : RealImagToComplex
  Sum : Sum  Inputs=|++  OutDataTypeStr=Inherit: Same as first input
  Sum1 : Sum  Inputs=|++
  Switch : Switch  Criteria=u2 ~= 0
  stop_out : Outport  VectorParamsAs1DForOutWhenUnconnected=off
  z_out : Outport  Port=2  VectorParamsAs1DForOutWhenUnconnected=off
  c_out : Outport  Port=3  VectorParamsAs1DForOutWhenUnconnected=off
  i_out : Outport  Port=4  VectorParamsAs1DForOutWhenUnconnected=off
  wires:
  i_in/1 -> Switch/1, Sum1/1
  c_in/1 -> c_out/1, Sum/2
  z_in/1 -> Complex to Real-Imag/1
  stop_in/1 -> Logical Operator/1
  Add/1 -> Compare To Constant/1
  Add1/1 -> Real-Imag to Complex/1
  Compare To Constant/1 -> Logical Operator/2
  Complex to Real-Imag/2 -> Product3/2, Product2/1, Product2/2
  Complex to Real-Imag/1 -> Product3/1, Product1/1, Product1/2
  Constant/1 -> Sum1/2
  Data Type Conversion2/1 -> z_out/1
  Gain/1 -> Real-Imag to Complex/2
  Logical Operator/1 -> stop_out/1, Switch/2
  Product1/1 -> Add1/1, Add/1
  Product2/1 -> Add1/2, Add/2
  Product3/1 -> Gain/1
  Real-Imag to Complex/1 -> Sum/1
  Sum/1 -> Data Type Conversion2/1
  Sum1/1 -> Switch/3
  Switch/1 -> i_out/1

== system gm_mandelbrot_fpga/mandelbrot_top/mandelbrot_core/mandelbroot_pipeline/mandelbroot_array_instance72 ==
  stop_in : Inport  OutDataTypeStr=boolean  PortDimensions=1  SampleTime=1.35e-08
  z_in : Inport  Port=2  OutDataTypeStr=fixdt(1, 18, 15)  PortDimensions=1  SampleTime=1.35e-08
      settings: SignalType=complex
  c_in : Inport  Port=3  OutDataTypeStr=fixdt(1, 18, 15)  PortDimensions=1  SampleTime=1.35e-08
      settings: SignalType=complex
  i_in : Inport  Port=4  OutDataTypeStr=fixdt(0, 7, 0)  PortDimensions=1  SampleTime=1.35e-08
  Add : Sum
  Add1 : Sum  Inputs=+-  OutDataTypeStr=Inherit: Same as first input
  Compare To Constant : simulink/Logic and Bit Operations/Compare To Constant  relop=>=  const=4  OutDataTypeStr=boolean
  Complex to Real-Imag : ComplexToRealImag
  Constant : Constant  OutDataTypeStr=uint8  SampleTime=-1
  Data Type Conversion2 : DataTypeConversion
  Gain : Gain  Gain=2  OutDataTypeStr=Inherit: Same as input  ParamDataTypeStr=Inherit: Same as input
  Logical Operator : Logic  Operator=OR  IconShape=distinctive  AllPortsSameDT=off  OutDataTypeStr=boolean
  Product1 : Product
  Product2 : Product
  Product3 : Product
  Real-Imag to Complex : RealImagToComplex
  Sum : Sum  Inputs=|++  OutDataTypeStr=Inherit: Same as first input
  Sum1 : Sum  Inputs=|++
  Switch : Switch  Criteria=u2 ~= 0
  stop_out : Outport  VectorParamsAs1DForOutWhenUnconnected=off
  z_out : Outport  Port=2  VectorParamsAs1DForOutWhenUnconnected=off
  c_out : Outport  Port=3  VectorParamsAs1DForOutWhenUnconnected=off
  i_out : Outport  Port=4  VectorParamsAs1DForOutWhenUnconnected=off
  wires:
  i_in/1 -> Switch/1, Sum1/1
  c_in/1 -> c_out/1, Sum/2
  z_in/1 -> Complex to Real-Imag/1
  stop_in/1 -> Logical Operator/1
  Add/1 -> Compare To Constant/1
  Add1/1 -> Real-Imag to Complex/1
  Compare To Constant/1 -> Logical Operator/2
  Complex to Real-Imag/2 -> Product3/2, Product2/1, Product2/2
  Complex to Real-Imag/1 -> Product3/1, Product1/1, Product1/2
  Constant/1 -> Sum1/2
  Data Type Conversion2/1 -> z_out/1
  Gain/1 -> Real-Imag to Complex/2
  Logical Operator/1 -> stop_out/1, Switch/2
  Product1/1 -> Add1/1, Add/1
  Product2/1 -> Add1/2, Add/2
  Product3/1 -> Gain/1
  Real-Imag to Complex/1 -> Sum/1
  Sum/1 -> Data Type Conversion2/1
  Sum1/1 -> Switch/3
  Switch/1 -> i_out/1

== system gm_mandelbrot_fpga/mandelbrot_top/mandelbrot_core/mandelbroot_pipeline/mandelbroot_array_instance73 ==
  stop_in : Inport  OutDataTypeStr=boolean  PortDimensions=1  SampleTime=1.35e-08
  z_in : Inport  Port=2  OutDataTypeStr=fixdt(1, 18, 15)  PortDimensions=1  SampleTime=1.35e-08
      settings: SignalType=complex
  c_in : Inport  Port=3  OutDataTypeStr=fixdt(1, 18, 15)  PortDimensions=1  SampleTime=1.35e-08
      settings: SignalType=complex
  i_in : Inport  Port=4  OutDataTypeStr=fixdt(0, 7, 0)  PortDimensions=1  SampleTime=1.35e-08
  Add : Sum
  Add1 : Sum  Inputs=+-  OutDataTypeStr=Inherit: Same as first input
  Compare To Constant : simulink/Logic and Bit Operations/Compare To Constant  relop=>=  const=4  OutDataTypeStr=boolean
  Complex to Real-Imag : ComplexToRealImag
  Constant : Constant  OutDataTypeStr=uint8  SampleTime=-1
  Data Type Conversion2 : DataTypeConversion
  Gain : Gain  Gain=2  OutDataTypeStr=Inherit: Same as input  ParamDataTypeStr=Inherit: Same as input
  Logical Operator : Logic  Operator=OR  IconShape=distinctive  AllPortsSameDT=off  OutDataTypeStr=boolean
  Product1 : Product
  Product2 : Product
  Product3 : Product
  Real-Imag to Complex : RealImagToComplex
  Sum : Sum  Inputs=|++  OutDataTypeStr=Inherit: Same as first input
  Sum1 : Sum  Inputs=|++
  Switch : Switch  Criteria=u2 ~= 0
  stop_out : Outport  VectorParamsAs1DForOutWhenUnconnected=off
  z_out : Outport  Port=2  VectorParamsAs1DForOutWhenUnconnected=off
  c_out : Outport  Port=3  VectorParamsAs1DForOutWhenUnconnected=off
  i_out : Outport  Port=4  VectorParamsAs1DForOutWhenUnconnected=off
  wires:
  i_in/1 -> Switch/1, Sum1/1
  c_in/1 -> c_out/1, Sum/2
  z_in/1 -> Complex to Real-Imag/1
  stop_in/1 -> Logical Operator/1
  Add/1 -> Compare To Constant/1
  Add1/1 -> Real-Imag to Complex/1
  Compare To Constant/1 -> Logical Operator/2
  Complex to Real-Imag/2 -> Product3/2, Product2/1, Product2/2
  Complex to Real-Imag/1 -> Product3/1, Product1/1, Product1/2
  Constant/1 -> Sum1/2
  Data Type Conversion2/1 -> z_out/1
  Gain/1 -> Real-Imag to Complex/2
  Logical Operator/1 -> stop_out/1, Switch/2
  Product1/1 -> Add1/1, Add/1
  Product2/1 -> Add1/2, Add/2
  Product3/1 -> Gain/1
  Real-Imag to Complex/1 -> Sum/1
  Sum/1 -> Data Type Conversion2/1
  Sum1/1 -> Switch/3
  Switch/1 -> i_out/1

== system gm_mandelbrot_fpga/mandelbrot_top/mandelbrot_core/mandelbroot_pipeline/mandelbroot_array_instance74 ==
  stop_in : Inport  OutDataTypeStr=boolean  PortDimensions=1  SampleTime=1.35e-08
  z_in : Inport  Port=2  OutDataTypeStr=fixdt(1, 18, 15)  PortDimensions=1  SampleTime=1.35e-08
      settings: SignalType=complex
  c_in : Inport  Port=3  OutDataTypeStr=fixdt(1, 18, 15)  PortDimensions=1  SampleTime=1.35e-08
      settings: SignalType=complex
  i_in : Inport  Port=4  OutDataTypeStr=fixdt(0, 7, 0)  PortDimensions=1  SampleTime=1.35e-08
  Add : Sum
  Add1 : Sum  Inputs=+-  OutDataTypeStr=Inherit: Same as first input
  Compare To Constant : simulink/Logic and Bit Operations/Compare To Constant  relop=>=  const=4  OutDataTypeStr=boolean
  Complex to Real-Imag : ComplexToRealImag
  Constant : Constant  OutDataTypeStr=uint8  SampleTime=-1
  Data Type Conversion2 : DataTypeConversion
  Gain : Gain  Gain=2  OutDataTypeStr=Inherit: Same as input  ParamDataTypeStr=Inherit: Same as input
  Logical Operator : Logic  Operator=OR  IconShape=distinctive  AllPortsSameDT=off  OutDataTypeStr=boolean
  Product1 : Product
  Product2 : Product
  Product3 : Product
  Real-Imag to Complex : RealImagToComplex
  Sum : Sum  Inputs=|++  OutDataTypeStr=Inherit: Same as first input
  Sum1 : Sum  Inputs=|++
  Switch : Switch  Criteria=u2 ~= 0
  stop_out : Outport  VectorParamsAs1DForOutWhenUnconnected=off
  z_out : Outport  Port=2  VectorParamsAs1DForOutWhenUnconnected=off
  c_out : Outport  Port=3  VectorParamsAs1DForOutWhenUnconnected=off
  i_out : Outport  Port=4  VectorParamsAs1DForOutWhenUnconnected=off
  wires:
  i_in/1 -> Switch/1, Sum1/1
  c_in/1 -> c_out/1, Sum/2
  z_in/1 -> Complex to Real-Imag/1
  stop_in/1 -> Logical Operator/1
  Add/1 -> Compare To Constant/1
  Add1/1 -> Real-Imag to Complex/1
  Compare To Constant/1 -> Logical Operator/2
  Complex to Real-Imag/2 -> Product3/2, Product2/1, Product2/2
  Complex to Real-Imag/1 -> Product3/1, Product1/1, Product1/2
  Constant/1 -> Sum1/2
  Data Type Conversion2/1 -> z_out/1
  Gain/1 -> Real-Imag to Complex/2
  Logical Operator/1 -> stop_out/1, Switch/2
  Product1/1 -> Add1/1, Add/1
  Product2/1 -> Add1/2, Add/2
  Product3/1 -> Gain/1
  Real-Imag to Complex/1 -> Sum/1
  Sum/1 -> Data Type Conversion2/1
  Sum1/1 -> Switch/3
  Switch/1 -> i_out/1

== system gm_mandelbrot_fpga/mandelbrot_top/mandelbrot_core/mandelbroot_pipeline/mandelbroot_array_instance75 ==
  stop_in : Inport  OutDataTypeStr=boolean  PortDimensions=1  SampleTime=1.35e-08
  z_in : Inport  Port=2  OutDataTypeStr=fixdt(1, 18, 15)  PortDimensions=1  SampleTime=1.35e-08
      settings: SignalType=complex
  c_in : Inport  Port=3  OutDataTypeStr=fixdt(1, 18, 15)  PortDimensions=1  SampleTime=1.35e-08
      settings: SignalType=complex
  i_in : Inport  Port=4  OutDataTypeStr=fixdt(0, 7, 0)  PortDimensions=1  SampleTime=1.35e-08
  Add : Sum
  Add1 : Sum  Inputs=+-  OutDataTypeStr=Inherit: Same as first input
  Compare To Constant : simulink/Logic and Bit Operations/Compare To Constant  relop=>=  const=4  OutDataTypeStr=boolean
  Complex to Real-Imag : ComplexToRealImag
  Constant : Constant  OutDataTypeStr=uint8  SampleTime=-1
  Data Type Conversion2 : DataTypeConversion
  Gain : Gain  Gain=2  OutDataTypeStr=Inherit: Same as input  ParamDataTypeStr=Inherit: Same as input
  Logical Operator : Logic  Operator=OR  IconShape=distinctive  AllPortsSameDT=off  OutDataTypeStr=boolean
  Product1 : Product
  Product2 : Product
  Product3 : Product
  Real-Imag to Complex : RealImagToComplex
  Sum : Sum  Inputs=|++  OutDataTypeStr=Inherit: Same as first input
  Sum1 : Sum  Inputs=|++
  Switch : Switch  Criteria=u2 ~= 0
  stop_out : Outport  VectorParamsAs1DForOutWhenUnconnected=off
  z_out : Outport  Port=2  VectorParamsAs1DForOutWhenUnconnected=off
  c_out : Outport  Port=3  VectorParamsAs1DForOutWhenUnconnected=off
  i_out : Outport  Port=4  VectorParamsAs1DForOutWhenUnconnected=off
  wires:
  i_in/1 -> Switch/1, Sum1/1
  c_in/1 -> c_out/1, Sum/2
  z_in/1 -> Complex to Real-Imag/1
  stop_in/1 -> Logical Operator/1
  Add/1 -> Compare To Constant/1
  Add1/1 -> Real-Imag to Complex/1
  Compare To Constant/1 -> Logical Operator/2
  Complex to Real-Imag/2 -> Product3/2, Product2/1, Product2/2
  Complex to Real-Imag/1 -> Product3/1, Product1/1, Product1/2
  Constant/1 -> Sum1/2
  Data Type Conversion2/1 -> z_out/1
  Gain/1 -> Real-Imag to Complex/2
  Logical Operator/1 -> stop_out/1, Switch/2
  Product1/1 -> Add1/1, Add/1
  Product2/1 -> Add1/2, Add/2
  Product3/1 -> Gain/1
  Real-Imag to Complex/1 -> Sum/1
  Sum/1 -> Data Type Conversion2/1
  Sum1/1 -> Switch/3
  Switch/1 -> i_out/1
